simulink model "Part2sm_lab4_2020b"  (R2020b)
settings: Solver=VariableStepAuto  StartTime=0.0  StopTime=20  RelTol=1e-3
undefined symbols (not defined in the file): l1, l2, l3, m1, m2, m3, X, Y, Z
libraries: nesl_utility x16, sm_lib x14
settings Model: Creator=Alex  LastModifiedBy=Alex
settings DebuggingCC: SFMachineParentedDataDiag=error

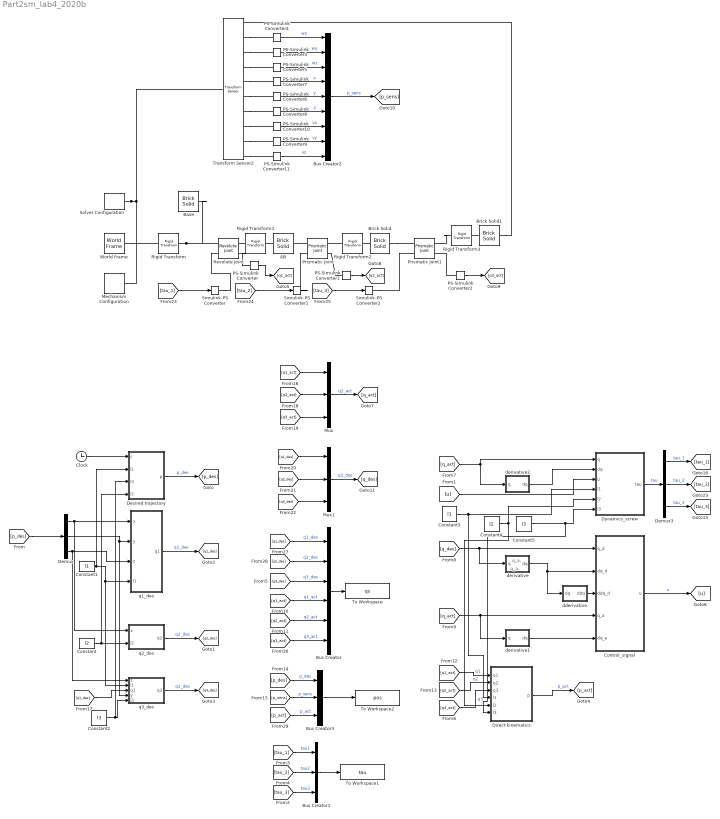
== system Part2sm_lab4_2020b ==
  note: q_a,
  note: q_a,
  AB : sm_lib/Body Elements/Brick Solid  GraphicAmbientColor=[0.15 0.15 0.15 1.0]  BasedOnType=Mass  BrickDimensions=AB  BrickDimensionUnits=m  CenterOfMass=[0 0 0]  CenterOfMassUnits=m  GraphicDiffuseColor=[0.5 0.5 0.5]  Density=1000  DensityUnits=kg/m^3  DoExposeReferenceFrame=off  GraphicEmissiveColor=[0.0 0.0 0.0 1.0]  ExportEntireGeometry=off  SerializedFrames=<Frames><Frame><Id>Frame1</Id><Value><Name>F1</Name><Origin><Source>GeometricFeature</Source><FeatureName>-z surface</FeatureName></Origin><PrimaryAxis><DefinedDirection>+Z</DefinedDirection><Source>ReferenceFrame</Source><SourceDirection>+Z</SourceDirection><FeatureName></FeatureName></PrimaryAxis><SecondaryAxis><DefinedDirection>-X</DefinedDirection><Source>ReferenceFrame</Source><SourceDirection>+X</SourceDirection><FeatureName></FeatureName></SecondaryAxis></Value></Frame><Frame><Id>Frame2</Id><Value><Name>F2</Name><Origin><Source>GeometricFeature</Source><FeatureName>+z surface</FeatureName></Origin><PrimaryAxis><DefinedDirection>+Z</DefinedDirection><Source>ReferenceFrame</Source><SourceDirection>-X</SourceDirection><FeatureName></FeatureName></PrimaryAxis><SecondaryAxis><DefinedDirection>+Y</DefinedDirection><Source>ReferenceFrame</Source><SourceDirection>+Y</SourceDirection><FeatureName></FeatureName></SecondaryAxis></Value></Frame></Frames>  MarkerShape=Sphere  MarkerSize=10  GraphicType=FromGeometry  InertiaType=CalculateFromGeometry  Mass=m1  MassUnits=kg  MomentsOfInertia=[1 1 1]  MomentsOfInertiaUnits=kg*m^2  GraphicOpacity=1.0  ProductsOfInertia=[0 0 0]  ProductsOfInertiaUnits=kg*m^2  GraphicShininess=75  GraphicSpecularColor=[0.5 0.5 0.5 1.0]  GraphicVisPropType=SimpleVisualProperties
  Base : sm_lib/Body Elements/Brick Solid  GraphicAmbientColor=[0.15 0.15 0.15 1.0]  BasedOnType=Density  BrickDimensions=Base  BrickDimensionUnits=m  CenterOfMass=[0 0 0]  CenterOfMassUnits=m  GraphicDiffuseColor=[0.5 0.5 0.5]  Density=1000  DensityUnits=kg/m^3  DoExposeReferenceFrame=on  GraphicEmissiveColor=[0.0 0.0 0.0 1.0]  ExportEntireGeometry=off  SerializedFrames=<Frames/>  MarkerShape=Sphere  MarkerSize=10  GraphicType=FromGeometry  InertiaType=CalculateFromGeometry  Mass=1  MassUnits=kg  MomentsOfInertia=[1 1 1]  MomentsOfInertiaUnits=kg*m^2  GraphicOpacity=1.0  ProductsOfInertia=[0 0 0]  ProductsOfInertiaUnits=kg*m^2  GraphicShininess=75  GraphicSpecularColor=[0.5 0.5 0.5 1.0]  GraphicVisPropType=SimpleVisualProperties
  Brick Solid : sm_lib/Body Elements/Brick Solid  GraphicAmbientColor=[0.15 0.15 0.15 1.0]  BasedOnType=Mass  BrickDimensions=BC  BrickDimensionUnits=m  CenterOfMass=[0 0 0]  CenterOfMassUnits=m  GraphicDiffuseColor=[0.5 0.5 0.5]  Density=1000  DensityUnits=kg/m^3  DoExposeReferenceFrame=off  GraphicEmissiveColor=[0.0 0.0 0.0 1.0]  ExportEntireGeometry=off  SerializedFrames=<Frames><Frame><Id>Frame1</Id><Value><Name>F1</Name><Origin><Source>GeometricFeature</Source><FeatureName>-x surface</FeatureName></Origin><PrimaryAxis><DefinedDirection>+Z</DefinedDirection><Source>ReferenceFrame</Source><SourceDirection>+X</SourceDirection><FeatureName></FeatureName></PrimaryAxis><SecondaryAxis><DefinedDirection>+Y</DefinedDirection><Source>ReferenceFrame</Source><SourceDirection>+Y</SourceDirection><FeatureName></FeatureName></SecondaryAxis></Value></Frame><Frame><Id>Frame2</Id><Value><Name>F2</Name><Origin><Source>GeometricFeature</Source><FeatureName>+x surface</FeatureName></Origin><PrimaryAxis><DefinedDirection>+Z</DefinedDirection><Source>ReferenceFrame</Source><SourceDirection>-Z</SourceDirection><FeatureName></FeatureName></PrimaryAxis><SecondaryAxis><DefinedDirection>+Y</DefinedDirection><Source>ReferenceFrame</Source><SourceDirection>+Y</SourceDirection><FeatureName></FeatureName></SecondaryAxis></Value></Frame></Frames>  MarkerShape=Sphere  MarkerSize=10  GraphicType=FromGeometry  InertiaType=CalculateFromGeometry  Mass=m2  MassUnits=kg  MomentsOfInertia=[1 1 1]  MomentsOfInertiaUnits=kg*m^2  GraphicOpacity=1.0  ProductsOfInertia=[0 0 0]  ProductsOfInertiaUnits=kg*m^2  GraphicShininess=75  GraphicSpecularColor=[0.5 0.5 0.5 1.0]  GraphicVisPropType=SimpleVisualProperties
  Brick Solid1 : sm_lib/Body Elements/Brick Solid  GraphicAmbientColor=[0.15 0.15 0.15 1.0]  BasedOnType=Mass  BrickDimensions=CD  BrickDimensionUnits=m  CenterOfMass=[0 0 0]  CenterOfMassUnits=m  GraphicDiffuseColor=[0.5 0.5 0.5]  Density=1000  DensityUnits=kg/m^3  DoExposeReferenceFrame=off  GraphicEmissiveColor=[0.0 0.0 0.0 1.0]  ExportEntireGeometry=off  SerializedFrames=<Frames><Frame><Id>Frame1</Id><Value><Name>F1</Name><Origin><Source>GeometricFeature</Source><FeatureName>-z surface</FeatureName></Origin><PrimaryAxis><DefinedDirection>+Z</DefinedDirection><Source>ReferenceFrame</Source><SourceDirection>+Z</SourceDirection><FeatureName></FeatureName></PrimaryAxis><SecondaryAxis><DefinedDirection>+X</DefinedDirection><Source>ReferenceFrame</Source><SourceDirection>+X</SourceDirection><FeatureName></FeatureName></SecondaryAxis></Value></Frame><Frame><Id>Frame2</Id><Value><Name>F2</Name><Origin><Source>GeometricFeature</Source><FeatureName>+z surface</FeatureName></Origin><PrimaryAxis><DefinedDirection>+Z</DefinedDirection><Source>ReferenceFrame</Source><SourceDirection>+Z</SourceDirection><FeatureName></FeatureName></PrimaryAxis><SecondaryAxis><DefinedDirection>+X</DefinedDirection><Source>ReferenceFrame</Source><SourceDirection>+X</SourceDirection><FeatureName></FeatureName></SecondaryAxis></Value></Frame></Frames>  MarkerShape=Sphere  MarkerSize=10  GraphicType=FromGeometry  InertiaType=CalculateFromGeometry  Mass=m3  MassUnits=kg  MomentsOfInertia=[1 1 1]  MomentsOfInertiaUnits=kg*m^2  GraphicOpacity=1.0  ProductsOfInertia=[0 0 0]  ProductsOfInertiaUnits=kg*m^2  GraphicShininess=75  GraphicSpecularColor=[0.5 0.5 0.5 1.0]  GraphicVisPropType=SimpleVisualProperties
  Bus Creator : BusCreator  Inputs=6
  Bus Creator1 : BusCreator  Inputs=3
  Bus Creator2 : BusCreator  Inputs=9
  Bus Creator3 : BusCreator  Inputs=3
  Clock : Clock
  Constant : Constant  Value=l2
  Constant1 : Constant  Value=l1
  Constant2 : Constant  Value=l3
  Constant3 : Constant  Value=l1
  Constant4 : Constant  Value=l2
  Constant5 : Constant  Value=l3
  Control_signal : MATLAB Function  TreatAsAtomicUnit=on
  Demux : Demux  Outputs=3
  Demux3 : Demux  Outputs=3
  Desired trajectory : MATLAB Function  TreatAsAtomicUnit=on
  Direct kinematics : MATLAB Function  TreatAsAtomicUnit=on
  Dynamics_screw : MATLAB Function  TreatAsAtomicUnit=on
  Mechanism Configuration : sm_lib/Utilities/Mechanism Configuration  UniformGravity=Constant  GravityVector=[0 0 -9.80665]  GravityVectorUnits=m/s^2  GravityUnits=m/s^2  LinearizationDelta=0.001  JointModeTransitionNonlinearIterations=2
  Mux : Mux  Inputs=3
  Mux1 : Mux  Inputs=3
  PS-Simulink Converter : nesl_utility/PS-Simulink Converter  PhysicalDomain=network_engine_domain  SubClassName=ps_output  LeftPortType=input  RightPortType=output  PseudoPeriodic=off  Frequencies=[]  Unit=rad  AffineConversion=off
      settings: SourceProductBaseCode=PW,SS
  PS-Simulink Converter{1..2,6..8} (5 alike) : nesl_utility/PS-Simulink Converter  PhysicalDomain=network_engine_domain  SubClassName=ps_output  LeftPortType=input  RightPortType=output  PseudoPeriodic=off  Frequencies=[]  Unit=m  AffineConversion=off
      settings: SourceProductBaseCode=PW,SS
  PS-Simulink Converter10 : nesl_utility/PS-Simulink Converter  PhysicalDomain=network_engine_domain  SubClassName=ps_output  LeftPortType=input  RightPortType=output  PseudoPeriodic=off  Frequencies=[]  Unit=m/s  AffineConversion=off
      settings: SourceProductBaseCode=PW,SS
  PS-Simulink Converter11 : nesl_utility/PS-Simulink Converter  PhysicalDomain=network_engine_domain  SubClassName=ps_output  LeftPortType=input  RightPortType=output  PseudoPeriodic=off  Frequencies=[]  Unit=m/s  AffineConversion=off
      settings: SourceProductBaseCode=PW,SS
  PS-Simulink Converter3 : nesl_utility/PS-Simulink Converter  PhysicalDomain=network_engine_domain  SubClassName=ps_output  LeftPortType=input  RightPortType=output  PseudoPeriodic=off  Frequencies=[]  Unit=rad/s  AffineConversion=off
      settings: SourceProductBaseCode=PW,SS
  PS-Simulink Converter4 : nesl_utility/PS-Simulink Converter  PhysicalDomain=network_engine_domain  SubClassName=ps_output  LeftPortType=input  RightPortType=output  PseudoPeriodic=off  Frequencies=[]  Unit=rad/s  AffineConversion=off
      settings: SourceProductBaseCode=PW,SS
  PS-Simulink Converter5 : nesl_utility/PS-Simulink Converter  PhysicalDomain=network_engine_domain  SubClassName=ps_output  LeftPortType=input  RightPortType=output  PseudoPeriodic=off  Frequencies=[]  Unit=rad/s  AffineConversion=off
      settings: SourceProductBaseCode=PW,SS
  PS-Simulink Converter9 : nesl_utility/PS-Simulink Converter  PhysicalDomain=network_engine_domain  SubClassName=ps_output  LeftPortType=input  RightPortType=output  PseudoPeriodic=off  Frequencies=[]  Unit=m/s  AffineConversion=off
      settings: SourceProductBaseCode=PW,SS
  Prismatic Joint : sm_lib/Joints/Prismatic Joint  JointMode=Normal  SenseConstraintForce=off  SenseConstraintForceX=off  SenseConstraintForceY=off  SenseConstraintForceZ=off  SenseConstraintTorque=off  SenseConstraintTorqueX=off  SenseConstraintTorqueY=off  SenseConstraintTorqueZ=off  SenseTotalForce=off  SenseTotalForceX=off  SenseTotalForceY=off  SenseTotalForceZ=off  SenseTotalTorque=off  SenseTotalTorqueX=off  SenseTotalTorqueY=off  SenseTotalTorqueZ=off  CompositeWrenchDir=FollowerOnBase  CompositeWrenchFrame=BaseFrame  EquilibriumPosition=0  EquilibriumPositionUnits=m  SpringStiffness=0  SpringStiffnessUnits=N/m  DampingCoefficient=0  DampingCoefficientUnits=N/(m/s)  TorqueActuationMode=InputTorque  MotionActuationMode=ComputedMotion  SensePosition=on  SenseVelocity=off  SenseAcceleration=off  SenseTorqueForce=off  SenseLowerLimitTorqueForce=off  SenseUpperLimitTorqueForce=off  LowerLimitSpecify=on  LowerLimitBound=-l2/2  LowerLimitBoundUnits=m  LowerLimitStiffness=1e6  LowerLimitStiffnessUnits=N/m  LowerLimitDamping=1e3  LowerLimitDampingUnits=N/(m/s)  LowerLimitTransitionRegionWidth=1e-4  LowerLimitTransitionRegionWidthUnits=m  UpperLimitSpecify=on  UpperLimitBound=l2/2  UpperLimitBoundUnits=m  UpperLimitStiffness=1e6  UpperLimitStiffnessUnits=N/m  UpperLimitDamping=1e3  UpperLimitDampingUnits=N/(m/s)  UpperLimitTransitionRegionWidth=1e-4  UpperLimitTransitionRegionWidthUnits=m  PositionTargetSpecify=off  PositionTargetPriority=High  PositionTargetValue=0  PositionTargetValueUnits=m  VelocityTargetSpecify=off  VelocityTargetPriority=High  VelocityTargetValue=0  VelocityTargetValueUnits=m/s
  Prismatic Joint1 : sm_lib/Joints/Prismatic Joint  JointMode=Normal  SenseConstraintForce=off  SenseConstraintForceX=off  SenseConstraintForceY=off  SenseConstraintForceZ=off  SenseConstraintTorque=off  SenseConstraintTorqueX=off  SenseConstraintTorqueY=off  SenseConstraintTorqueZ=off  SenseTotalForce=off  SenseTotalForceX=off  SenseTotalForceY=off  SenseTotalForceZ=off  SenseTotalTorque=off  SenseTotalTorqueX=off  SenseTotalTorqueY=off  SenseTotalTorqueZ=off  CompositeWrenchDir=FollowerOnBase  CompositeWrenchFrame=BaseFrame  EquilibriumPosition=0  EquilibriumPositionUnits=m  SpringStiffness=0  SpringStiffnessUnits=N/m  DampingCoefficient=0  DampingCoefficientUnits=N/(m/s)  TorqueActuationMode=InputTorque  MotionActuationMode=ComputedMotion  SensePosition=on  SenseVelocity=off  SenseAcceleration=off  SenseTorqueForce=off  SenseLowerLimitTorqueForce=off  SenseUpperLimitTorqueForce=off  LowerLimitSpecify=on  LowerLimitBound=-l3/2  LowerLimitBoundUnits=m  LowerLimitStiffness=1e6  LowerLimitStiffnessUnits=N/m  LowerLimitDamping=1e3  LowerLimitDampingUnits=N/(m/s)  LowerLimitTransitionRegionWidth=1e-4  LowerLimitTransitionRegionWidthUnits=m  UpperLimitSpecify=on  UpperLimitBound=l3/2  UpperLimitBoundUnits=m  UpperLimitStiffness=1e6  UpperLimitStiffnessUnits=N/m  UpperLimitDamping=1e3  UpperLimitDampingUnits=N/(m/s)  UpperLimitTransitionRegionWidth=1e-4  UpperLimitTransitionRegionWidthUnits=m  PositionTargetSpecify=off  PositionTargetPriority=High  PositionTargetValue=0  PositionTargetValueUnits=m  VelocityTargetSpecify=off  VelocityTargetPriority=High  VelocityTargetValue=0  VelocityTargetValueUnits=m/s
  Revolute Joint : sm_lib/Joints/Revolute Joint  JointMode=Normal  SenseConstraintForce=off  SenseConstraintForceX=off  SenseConstraintForceY=off  SenseConstraintForceZ=off  SenseConstraintTorque=off  SenseConstraintTorqueX=off  SenseConstraintTorqueY=off  SenseConstraintTorqueZ=off  SenseTotalForce=off  SenseTotalForceX=off  SenseTotalForceY=off  SenseTotalForceZ=off  SenseTotalTorque=off  SenseTotalTorqueX=off  SenseTotalTorqueY=off  SenseTotalTorqueZ=off  CompositeWrenchDir=FollowerOnBase  CompositeWrenchFrame=BaseFrame  EquilibriumPosition=0  EquilibriumPositionUnits=deg  SpringStiffness=0  SpringStiffnessUnits=N*m/deg  DampingCoefficient=0  DampingCoefficientUnits=N*m/(deg/s)  TorqueActuationMode=InputTorque  MotionActuationMode=ComputedMotion  SensePosition=on  SenseVelocity=off  SenseAcceleration=off  SenseTorqueForce=off  SenseLowerLimitTorqueForce=off  SenseUpperLimitTorqueForce=off  LowerLimitSpecify=off  LowerLimitBound=-90  LowerLimitBoundUnits=deg  LowerLimitStiffness=1e4  LowerLimitStiffnessUnits=N*m/deg  LowerLimitDamping=10  LowerLimitDampingUnits=N*m/(deg/s)  LowerLimitTransitionRegionWidth=0.1  LowerLimitTransitionRegionWidthUnits=deg  UpperLimitSpecify=off  UpperLimitBound=90  UpperLimitBoundUnits=deg  UpperLimitStiffness=1e4  UpperLimitStiffnessUnits=N*m/deg  UpperLimitDamping=10  UpperLimitDampingUnits=N*m/(deg/s)  UpperLimitTransitionRegionWidth=0.1  UpperLimitTransitionRegionWidthUnits=deg  PositionTargetSpecify=off  PositionTargetPriority=High  PositionTargetValue=0  PositionTargetValueUnits=deg  VelocityTargetSpecify=off  VelocityTargetPriority=High  VelocityTargetValue=0  VelocityTargetValueUnits=deg/s
  Rigid Transform : sm_lib/Frames and Transforms/Rigid Transform  TranslationMethod=None  TranslationStandardOffset=0  TranslationLengthUnit=m  TranslationStandardAxis=+Z  TranslationCartesianOffset=[0 0 0]  TranslationROffset=0  TranslationROffsetUnits=m  TranslationZOffset=0  TranslationZOffsetUnits=m  TranslationThetaOffset=0  TranslationThetaOffsetUnits=deg  RotationMethod=StandardAxis  RotationAngleUnits=deg  RotationStandardAxis=-Y  RotationAngle=90  RotationArbitraryAxis=[0 0 1]  FollAlignAxisA=+X  BaseAlignAxisA=+Y  FollAlignAxisB=+Y  BaseAlignAxisB=+Z  RotationSequenceAxes=FollowerAxes  RotationSequence=XYX  RotationSequenceAngles=[0 0 0]  RotationSequenceAnglesUnits=deg  RotationMatrix=[1 0 0; 0 1 0; 0 0 1]
  Rigid Transform1 : sm_lib/Frames and Transforms/Rigid Transform  TranslationMethod=None  TranslationStandardOffset=0  TranslationLengthUnit=m  TranslationStandardAxis=+Z  TranslationCartesianOffset=[0 0 0]  TranslationROffset=0  TranslationROffsetUnits=m  TranslationZOffset=0  TranslationZOffsetUnits=m  TranslationThetaOffset=0  TranslationThetaOffsetUnits=deg  RotationMethod=StandardAxis  RotationAngleUnits=deg  RotationStandardAxis=+Y  RotationAngle=90  RotationArbitraryAxis=[0 0 1]  FollAlignAxisA=+X  BaseAlignAxisA=+Y  FollAlignAxisB=+Y  BaseAlignAxisB=+Z  RotationSequenceAxes=FollowerAxes  RotationSequence=XYX  RotationSequenceAngles=[0 0 0]  RotationSequenceAnglesUnits=deg  RotationMatrix=[1 0 0; 0 1 0; 0 0 1]
  Rigid Transform2 : sm_lib/Frames and Transforms/Rigid Transform  TranslationMethod=StandardAxis  TranslationStandardOffset=l2/2  TranslationLengthUnit=m  TranslationStandardAxis=-Z  TranslationCartesianOffset=[0 0 0]  TranslationROffset=0  TranslationROffsetUnits=m  TranslationZOffset=0  TranslationZOffsetUnits=m  TranslationThetaOffset=0  TranslationThetaOffsetUnits=deg  RotationMethod=None  RotationAngleUnits=deg  RotationStandardAxis=+Z  RotationAngle=0.0  RotationArbitraryAxis=[0 0 1]  FollAlignAxisA=+X  BaseAlignAxisA=+Y  FollAlignAxisB=+Y  BaseAlignAxisB=+Z  RotationSequenceAxes=FollowerAxes  RotationSequence=XYX  RotationSequenceAngles=[0 0 0]  RotationSequenceAnglesUnits=deg  RotationMatrix=[1 0 0; 0 1 0; 0 0 1]
  Rigid Transform3 : sm_lib/Frames and Transforms/Rigid Transform  TranslationMethod=StandardAxis  TranslationStandardOffset=l3/2  TranslationLengthUnit=m  TranslationStandardAxis=-Z  TranslationCartesianOffset=[0 0 0]  TranslationROffset=0  TranslationROffsetUnits=m  TranslationZOffset=0  TranslationZOffsetUnits=m  TranslationThetaOffset=0  TranslationThetaOffsetUnits=deg  RotationMethod=None  RotationAngleUnits=deg  RotationStandardAxis=+Z  RotationAngle=0.0  RotationArbitraryAxis=[0 0 1]  FollAlignAxisA=+X  BaseAlignAxisA=+Y  FollAlignAxisB=+Y  BaseAlignAxisB=+Z  RotationSequenceAxes=FollowerAxes  RotationSequence=XYX  RotationSequenceAngles=[0 0 0]  RotationSequenceAnglesUnits=deg  RotationMatrix=[1 0 0; 0 1 0; 0 0 1]
  Simulink-PS Converter : nesl_utility/Simulink-PS Converter  PhysicalDomain=network_engine_domain  SubClassName=ps_input  LeftPortType=input  RightPortType=output  PseudoPeriodic=off  Frequencies=[]  NoiseDistribution=none  NoiseParameters=[]  Unit=N*m  AffineConversion=off  FilteringAndDerivatives=provide  SimscapeFilterOrder=1  InputFilterTimeConstant=0.001  UdotUserProvided=0
      settings: SourceProductBaseCode=PW,SS
  Simulink-PS Converter1 : nesl_utility/Simulink-PS Converter  PhysicalDomain=network_engine_domain  SubClassName=ps_input  LeftPortType=input  RightPortType=output  PseudoPeriodic=off  Frequencies=[]  NoiseDistribution=none  NoiseParameters=[]  Unit=N  AffineConversion=off  FilteringAndDerivatives=provide  SimscapeFilterOrder=1  InputFilterTimeConstant=0.001  UdotUserProvided=0
      settings: SourceProductBaseCode=PW,SS
  Simulink-PS Converter2 : nesl_utility/Simulink-PS Converter  PhysicalDomain=network_engine_domain  SubClassName=ps_input  LeftPortType=input  RightPortType=output  PseudoPeriodic=off  Frequencies=[]  NoiseDistribution=none  NoiseParameters=[]  Unit=N  AffineConversion=off  FilteringAndDerivatives=provide  SimscapeFilterOrder=1  InputFilterTimeConstant=0.001  UdotUserProvided=0
      settings: SourceProductBaseCode=PW,SS
  Solver Configuration : nesl_utility/Solver Configuration  PhysicalDomain=network_engine_domain  SubClassName=solver  LeftPortType=input  RightPortType=generic  Tones=[]  Harmonics=[]  SimulateNoise=off  Profile=off  UseLocalSampling=off  EnableSwitchedLinearOptims=on  FrequencyDomain=off  UseCCode=off  RelTol=0.001  AbsTol=1e-06  MinStep=1e-09  ToWorkspace=off  RevertToSquareIcSolve=off  NumHomotopyIterations=100  PhasorMode=off  PhasorModeNumHarmonics=1  DoDC=off  ResidualTolerance=1e-09  UseLocalSolver=off  LocalSolverChoice=NE_BACKWARD_EULER_ADVANCER  LocalSolverSampleTime=0.001  DoFixedCost=off  MaxNonlinIter=3  MaxModeIter=2  ComputeImpulses=off  ImpulseIterations=2  LinearAlgebra=Sparse  EquationFormulation=NE_TIME_EF  DelaysMemoryBudget=1024  AutomaticFiltering=on  FilteringTimeConstant=0.001  PartitionStorageMethod=AS_NEEDED  PartitionMemoryBudget=1024  PartitionMethod=FAST
      settings: SourceProductBaseCode=PW,SS
  To Workspace : ToWorkspace  VariableName=qs  SaveFormat=Timeseries  SampleTime=-1
  To Workspace1 : ToWorkspace  VariableName=tau  SaveFormat=Timeseries  SampleTime=-1
  To Workspace2 : ToWorkspace  VariableName=pos  SaveFormat=Timeseries  SampleTime=-1
  Transform Sensor2 : sm_lib/Frames and Transforms/Transform Sensor  MeasurementFrame=Base  SenseAngle=off  SenseAxis=off  SenseAngle1=off  SenseAngle2=off  SenseAngle3=off  SenseQ=off  SenseR=off  SenseOmegaX=on  SenseOmegaY=on  SenseOmegaZ=on  SenseOmega1=off  SenseOmega2=off  SenseOmega3=off  SenseQDot=off  SenseRDot=off  SenseAlphaX=off  SenseAlphaY=off  SenseAlphaZ=off  SenseAlpha1=off  SenseAlpha2=off  SenseAlpha3=off  SenseQDDot=off  SenseRDDot=off  SenseX=on  SenseY=on  SenseZ=on  SenseRad=off  SenseAzim=off  SenseDist=off  SenseInc=off  SenseXDot=on  SenseYDot=on  SenseZDot=on  SenseRadDot=off  SenseAzimDot=off  SenseDistDot=off  SenseIncDot=off  SenseXDDot=off  SenseYDDot=off  SenseZDDot=off  SenseRadDDot=off  SenseAzimDDot=off  SenseDistDDot=off  SenseIncDDot=off
  World Frame : sm_lib/Frames and Transforms/World Frame
  dderivative : Subsystem
  derivative : Subsystem
  derivative1 : Subsystem
  derivative2 : Subsystem
  q1_des : MATLAB Function  TreatAsAtomicUnit=on
  q2_des : MATLAB Function  TreatAsAtomicUnit=on
  q3_des : MATLAB Function  TreatAsAtomicUnit=on
  wires:
  [q1_des] -> q3_des/3(q1)
  Desired trajectory/1(p) -> [p_des]  "p_des"
  PS-Simulink Converter8/1 -> Bus Creator2/6  "z"
  PS-Simulink Converter9/1 -> Bus Creator2/8  "vy"
  Constant2/1 -> Desired trajectory/3(l3), q3_des/5(l3)
  PS-Simulink Converter3/1 -> Bus Creator2/2  "wy"
  PS-Simulink Converter6/1 -> Bus Creator2/5  "y"
  PS-Simulink Converter4/1 -> Bus Creator2/1  "wx"
  PS-Simulink Converter7/1 -> Bus Creator2/4  "x"
  PS-Simulink Converter11/1 -> Bus Creator2/9  "vz"
  PS-Simulink Converter1/1 -> [q2_act]
  Bus Creator2/1 -> [p_sens]  "p_sens"
  Clock/1 -> Desired trajectory/1(t)
  PS-Simulink Converter2/1 -> [q3_act]
  PS-Simulink Converter/1 -> [q1_act]
  PS-Simulink Converter5/1 -> Bus Creator2/3  "wz"
  Constant/1 -> Desired trajectory/4(l2), q2_des/2(l2)
  Demux/1 -> q2_des/1(x), q1_des/1(x)
  q3_des/1(q3) -> [q3_des]  "q3_des"
  q2_des/1(q2) -> [q2_des]  "q2_des"
  Demux/3 -> q3_des/1(z), q1_des/3(z)
  Constant1/1 -> Desired trajectory/2(l1), q3_des/2(l1), q1_des/4(l1)
  Demux/2 -> q3_des/4(y), q1_des/2(y)
  q1_des/1(q1) -> [q1_des]  "q1_des"
  [p_des] -> Demux/1
  PS-Simulink Converter10/1 -> Bus Creator2/7  "vx"
  Demux3/1 -> [tau_1]  "tau_1"
  derivative2/1(dq) -> Dynamics_screw/2(dq)
  [q3_act] -> Direct kinematics/3(q3)  "q3"
  Demux3/3 -> [tau_3]  "tau_3"
  Demux3/2 -> [tau_2]  "tau_2"
  [q_act] -> Dynamics_screw/1(q), derivative2/1(q)
  derivative1/1(dq) -> Control_signal/5(dq_a)
  Direct kinematics/1(p) -> [p_act]  "p_act"
  [q_des] -> derivative/1(q), Control_signal/1(q_d)
  [q_act] -> Control_signal/4(q_a), derivative1/1(q)
  Control_signal/1(u) -> [u]  "u"
  dderivative/1(ddq) -> Control_signal/3(ddq_d)
  [q1_act] -> Direct kinematics/1(q1)  "q1"
  [u] -> Dynamics_screw/3(u)
  derivative/1(dq) -> dderivative/1(dq), Control_signal/2(dq_d)
  [q2_act] -> Direct kinematics/2(q2)  "q2"
  Dynamics_screw/1(tau) -> Demux3/1  "tau"
  [q3_act] -> Mux/3
  [q2_act] -> Mux/2
  [q1_act] -> Mux/1
  Mux/1 -> [q_act]  "q2_act"
  [q2_des] -> Mux1/2
  [q3_des] -> Mux1/3
  [q1_des] -> Mux1/1
  Mux1/1 -> [q_des]  "q2_des"
  Constant3/1 -> Direct kinematics/4(l1), Dynamics_screw/4(l1)
  Constant4/1 -> Direct kinematics/5(l2), Dynamics_screw/5(l2)
  Constant5/1 -> Direct kinematics/6(l3), Dynamics_screw/6(l3)
  [tau_1] -> Simulink-PS Converter/1
  [tau_2] -> Simulink-PS Converter1/1
  [tau_3] -> Simulink-PS Converter2/1
  Bus Creator3/1 -> To Workspace2/1
  [q3_act] -> Bus Creator/6  "q3_act"
  [p_sens] -> Bus Creator3/2  "p_sens"
  [q1_act] -> Bus Creator/4  "q1_act"
  [q1_des] -> Bus Creator/1  "q1_des"
  [p_des] -> Bus Creator3/1  "p_des"
  Bus Creator1/1 -> To Workspace1/1
  [tau_2] -> Bus Creator1/2  "tau2"
  [q2_des] -> Bus Creator/2  "q2_des"
  [tau_3] -> Bus Creator1/3  "tau3"
  [q3_des] -> Bus Creator/3  "q3_des"
  [q2_act] -> Bus Creator/5  "q2_act"
  Bus Creator/1 -> To Workspace/1
  [tau_1] -> Bus Creator1/1  "tau1"
  [p_act] -> Bus Creator3/3  "p_act"
  connections:
  Solver Configuration/RConn1 -- Rigid Transform/LConn1 -- World Frame/RConn1 -- Mechanism Configuration/RConn1 -- Transform Sensor2/LConn1
  Rigid Transform/RConn1 -- Revolute Joint/LConn1 -- Base/RConn1
  Rigid Transform3/LConn1 -- Prismatic Joint1/RConn1
  Brick Solid/RConn1 -- Prismatic Joint1/LConn1
  Transform Sensor2/RConn3 -- PS-Simulink Converter3/LConn1
  Rigid Transform2/LConn1 -- Prismatic Joint/RConn1
  Simulink-PS Converter2/RConn1 -- Prismatic Joint1/LConn2
  Transform Sensor2/RConn5 -- PS-Simulink Converter7/LConn1
  Revolute Joint/RConn2 -- PS-Simulink Converter/LConn1
  PS-Simulink Converter1/LConn1 -- Prismatic Joint/RConn2
  Brick Solid1/RConn1 -- Transform Sensor2/RConn1
  Transform Sensor2/RConn9 -- PS-Simulink Converter9/LConn1
  Transform Sensor2/RConn4 -- PS-Simulink Converter5/LConn1
  Transform Sensor2/RConn7 -- PS-Simulink Converter8/LConn1
  Transform Sensor2/RConn6 -- PS-Simulink Converter6/LConn1
  PS-Simulink Converter2/LConn1 -- Prismatic Joint1/RConn2
  Rigid Transform2/RConn1 -- Brick Solid/LConn1
  Simulink-PS Converter1/RConn1 -- Prismatic Joint/LConn2
  Rigid Transform1/LConn1 -- Revolute Joint/RConn1
  AB/LConn1 -- Rigid Transform1/RConn1
  Brick Solid1/LConn1 -- Rigid Transform3/RConn1
  Transform Sensor2/RConn8 -- PS-Simulink Converter10/LConn1
  Simulink-PS Converter/RConn1 -- Revolute Joint/LConn2
  Transform Sensor2/RConn10 -- PS-Simulink Converter11/LConn1
  Transform Sensor2/RConn2 -- PS-Simulink Converter4/LConn1
  Prismatic Joint/LConn1 -- AB/RConn1

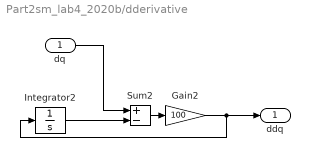
== system Part2sm_lab4_2020b/dderivative ==
  dq : Inport
  Gain2 : Gain  Gain=100
  Integrator2 : Integrator
  Sum2 : Sum  Inputs=+-
  ddq : Outport
  wires:
  dq/1 -> Sum2/1
  Integrator2/1 -> Sum2/2
  Sum2/1 -> Gain2/1
  Gain2/1 -> ddq/1, Integrator2/1

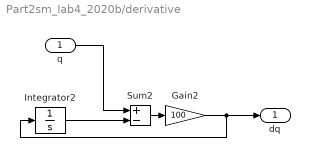
== system Part2sm_lab4_2020b/derivative ==
  q : Inport
  Gain2 : Gain  Gain=100
  Integrator2 : Integrator
  Sum2 : Sum  Inputs=+-
  dq : Outport
  wires:
  q/1 -> Sum2/1
  Integrator2/1 -> Sum2/2
  Sum2/1 -> Gain2/1
  Gain2/1 -> dq/1, Integrator2/1

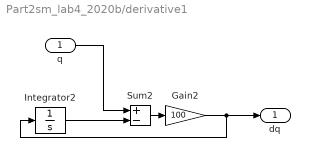
== system Part2sm_lab4_2020b/derivative1 ==
  q : Inport
  Gain2 : Gain  Gain=100
  Integrator2 : Integrator
  Sum2 : Sum  Inputs=+-
  dq : Outport
  wires:
  q/1 -> Sum2/1
  Integrator2/1 -> Sum2/2
  Sum2/1 -> Gain2/1
  Gain2/1 -> dq/1, Integrator2/1

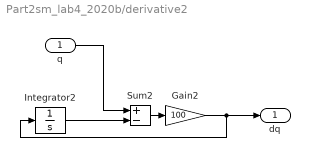
== system Part2sm_lab4_2020b/derivative2 ==
  q : Inport
  Gain2 : Gain  Gain=100
  Integrator2 : Integrator
  Sum2 : Sum  Inputs=+-
  dq : Outport
  wires:
  q/1 -> Sum2/1
  Integrator2/1 -> Sum2/2
  Sum2/1 -> Gain2/1
  Gain2/1 -> dq/1, Integrator2/1

== matlab function Part2sm_lab4_2020b/q1_des ==
  data: x input; q1 output; y input; z input; l1 input
function q1 = fcn(x,y,z,l1)

q1 = atan2(z,-y)-pi/2;

end

== matlab function Part2sm_lab4_2020b/Desired trajectory ==
  data: p output; t input; l1 input; l3 input; l2 input
function p = fcn(t, l1,l3,l2)
p = [l3/8*cos(t)+l2/2
    t/100
    l3/8*sin(t)+l1+l3/2];

== matlab function Part2sm_lab4_2020b/q2_des ==
  data: x input; q2 output; l2 input
function q2 = fcn(x,l2)
q2 = x - l2/2;
end

== matlab function Part2sm_lab4_2020b/q3_des ==
  data: z input; q3 output; l1 input; q1 input; y input; l3 input
function q3 = fcn(z,l1, q1,y,l3)
q3 = z/sin(atan2(z,-y))-l1-l3/2;
end

== matlab function Part2sm_lab4_2020b/Control_signal ==
  data: q_d input; dq_d input; u output; ddq_d input; q_a input; dq_a input
function u = fcn(q_d,dq_d,ddq_d, q_a,dq_a)
Ka=10;
Kv=10;
Kp=150;
u = Ka*ddq_d + Kv*(dq_d-dq_a) + Kp*(q_d-q_a);

== matlab function Part2sm_lab4_2020b/Dynamics_screw ==
  data: q input; dq input; u input; tau output; l1 input; l2 input; l3 input
function tau= fcn(q,dq,u,l1,l2,l3)
q1 = [1 0 0]*q;
q2 = [0 1 0]*q;
q3 = [0 0 1]*q;
m1 = 6.287;
m2 = 17.506;
m3 = 6.494; 
g=9.80665; 
jx1 =0.10848;
jy1 =0.10848;
jz1=0.00477419;

jx2 = 4.34838e-05;
jy2 = 0.000988048;
jz2 = 0.000988048;

jx3 = 0.0433821;
jy3 = 0.0433821;
jz3 = 0.00190924;

M =[jx1 + jx2 + jx3 + (l1^2*m1)/4 + l1^2*m2 + l1^2*m3 + m3*q3^2 + 2*l1*m3*q3, 0, 0
    0, m2 + m3, 0
    0, 0, m3];
 
C =[ -m3*(l1 + q3)
    0
    0];
 
N =[ - (g*sin(q1)*(l1*m1 + 2*l1*m2 + 2*l1*m3 + 2*m3*q3))/2
    0
    g*m3*cos(q1)];
tau=M*u+C .* dq + N;

== matlab function Part2sm_lab4_2020b/Direct kinematics ==
  data: q1 input; p output; q2 input; q3 input; l1 input; l2 input; l3 input
function p = fcn(q1, q2, q3,l1,l2,l3)
% direct kinematics
p = [l2/2 + q2
    sin(q1)*(l1 + l3/2 + q3)
    cos(q1)*(l1+l3/2+q3)
    1];
